simulink model "EX_Gain_2mdl"  (Simulink 4.00)
settings: Solver=ode45  StartTime=0.0  StopTime=10.0  RelTol=1e-3
settings Model: LastModifiedBy=Администратор

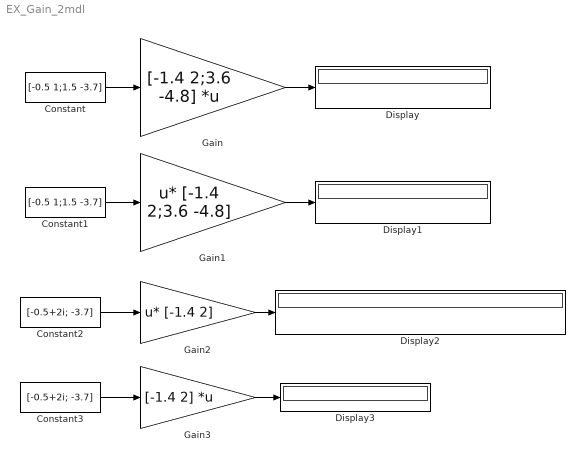
== system EX_Gain_2mdl ==
  Constant : Constant  Value=[-0.5 1;1.5 -3.7]  VectorParams1D=off
  Constant1 : Constant  Value=[-0.5 1;1.5 -3.7]  VectorParams1D=off
  Constant2 : Constant  Value=[-0.5+2i; -3.7]  VectorParams1D=off
  Constant3 : Constant  Value=[-0.5+2i; -3.7]  VectorParams1D=off
  Display{,1..3} (4 alike) : Display
      settings: Format=short
  Gain : Gain  Gain=[-1.4 2;3.6 -4.8]  Multiplication=Matrix(K*u)  SaturateOnIntegerOverflow=on
  Gain1 : Gain  Gain=[-1.4 2;3.6 -4.8]  Multiplication=Matrix(u*K)  SaturateOnIntegerOverflow=on
  Gain2 : Gain  Gain=[-1.4 2]  Multiplication=Matrix(u*K)  SaturateOnIntegerOverflow=on
  Gain3 : Gain  Gain=[-1.4 2]  Multiplication=Matrix(K*u)  SaturateOnIntegerOverflow=on
  wires:
  Constant/1 -> Gain/1
  Gain/1 -> Display/1
  Constant1/1 -> Gain1/1
  Gain1/1 -> Display1/1
  Constant2/1 -> Gain2/1
  Gain2/1 -> Display2/1
  Constant3/1 -> Gain3/1
  Gain3/1 -> Display3/1
